simulink model "VEHICLESUSPENSION"  (R2023b)
settings: Solver=VariableStepAuto  StartTime=0.0  StopTime=69  RelTol=1e-3
values from neighbouring files (symbols this model uses):
  A = [0 1 0 0 ... (first row only)    [vehicles_uspension.m]
  B = [0;k1/m1;0;0]    [vehicles_uspension.m]
  C = [0 0 1 0]    [vehicles_uspension.m]
  K = lqr(a_bar,b_bar,q,r)    [vehicles_uspension.m]
settings Model: LastModifiedBy=91798

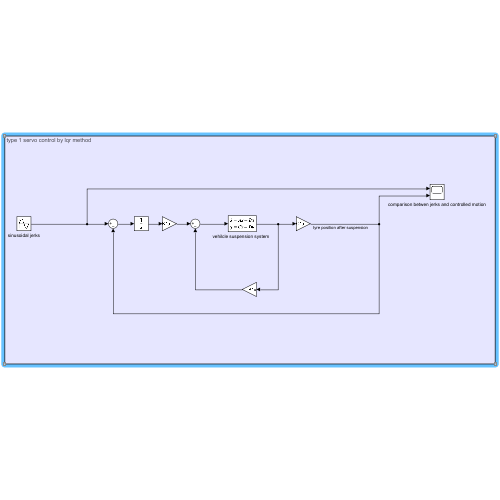
[thumbnail: Simulink's stored preview of the top-level diagram]
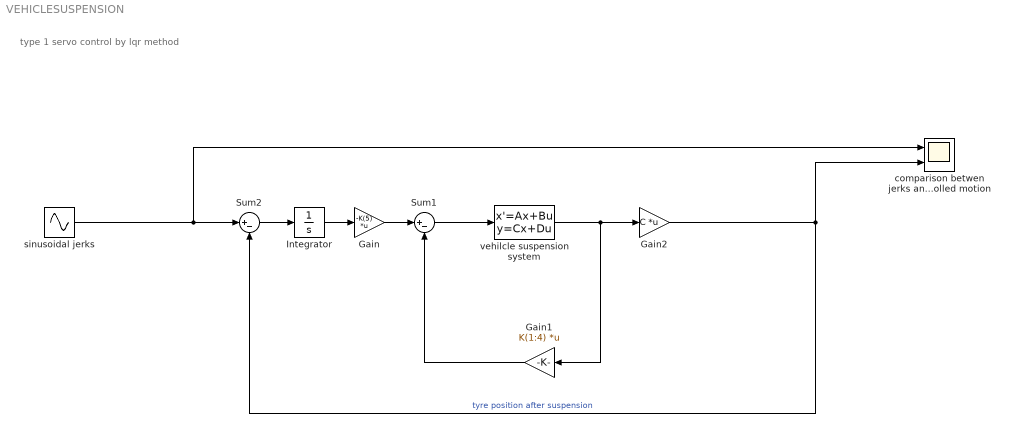
== system VEHICLESUSPENSION ==
  note: type 1 servo control by lqr method
  Gain : Gain  Gain=-K(5)  Multiplication=Matrix(K*u)
  Gain1 : Gain  Gain=K(1:4)  Multiplication=Matrix(K*u)
  Gain2 : Gain  Gain=C  Multiplication=Matrix(K*u)
  Integrator : Integrator
  Sum1 : Sum  Inputs=|+-
  Sum2 : Sum  Inputs=|+-
  comparison betwen jerks and controlled motion : Scope  NumInputPorts=2
  sinusoidal jerks : Sin  SampleTime=0
  "vehilcle suspension system  " : StateSpace  A=A  B=B  C=eye(4)  D=zeros(4,1)  InitialCondition=0
  wires:
  Gain1/1 -> Sum1/2
  Sum1/1 -> "vehilcle suspension system  "/1
  "vehilcle suspension system  "/1 -> Gain1/1, Gain2/1
  Gain2/1 -> comparison betwen jerks and controlled motion/2, Sum2/2  "tyre position after suspension"
  Gain/1 -> Sum1/1
  Sum2/1 -> Integrator/1
  Integrator/1 -> Gain/1
  sinusoidal jerks/1 -> comparison betwen jerks and controlled motion/1, Sum2/1
